simulink model "active_suspension"  (R2017a)
settings: Solver=VariableStepAuto  StartTime=0.0  StopTime=10.0  RelTol=1e-3
values from neighbouring files (symbols this model uses):
  A = z^2+den{1}(2)*z + den{1}(3)    [abs_spring18.m]    (also in active_suspension_ss.m = [0                 1                0                     0; active_suspension_ss_R.m = [0                 1                0                     0; active_suspension_ss_spring18.m = [0                 1                0                     0; double_integrator_deadbeat.m = [0 1; 0 0])
  B = num{1}(1)*z^2 + num{1}(2)*z + num{1}(3)    [abs_spring18.m]    (also in active_suspension_ss.m = [0                 0; active_suspension_ss_R.m = [0                 0; active_suspension_ss_spring18.m = [0                 0; double_integrator_deadbeat.m = [0;1])
  h = 0.05    [BLDC_partial2_fall18.m]    (also in abs_spring18.m = 0.2; active_suspension_ss.m = 0.00416985950901; active_suspension_ss_R.m = 0.00416985950901; active_suspension_ss_spring18.m = 0.004)
  L = acker(Phi, Gamma_u, p_d)    [active_suspension_ss_spring18.m]    (also in double_integrator_deadbeat.m = L'; final_dummy.m = Asf\bsf; hw_tank_simulink_pid_tuning.m = 2.84722131148; maglev_ss_partial2_spring18.m = place(A, B, pc))
undefined symbols (not defined in the file or in its folder): Lsh
settings Model: Creator=kjartan  LastModifiedBy=kjartan

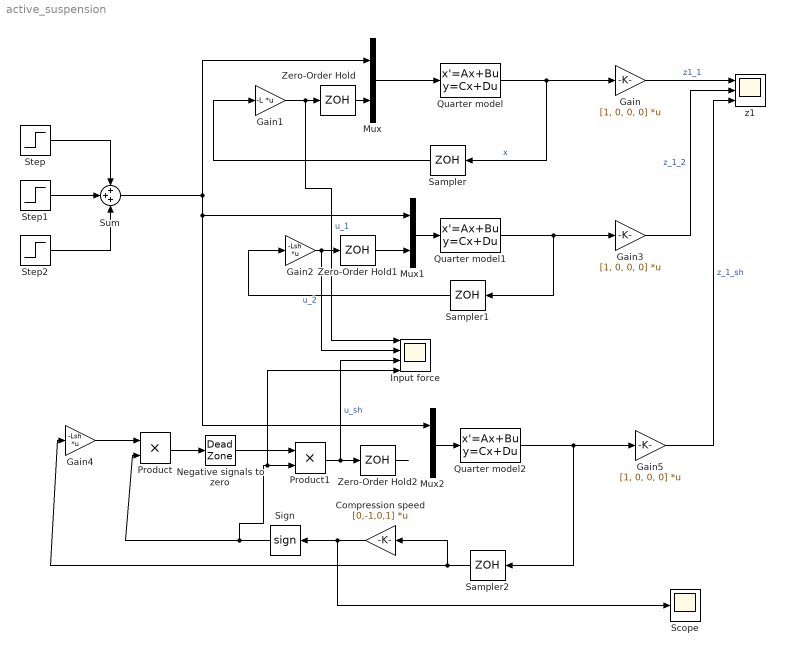
== system active_suspension ==
  Compression speed : Gain  Gain=[0,-1,0,1]  Multiplication=Matrix(K*u)
  Gain : Gain  Gain=[1, 0, 0, 0]  Multiplication=Matrix(K*u)
  Gain1 : Gain  Gain=-L  Multiplication=Matrix(K*u)
  Gain2 : Gain  Gain=-Lsh  Multiplication=Matrix(K*u)
  Gain3 : Gain  Gain=[1, 0, 0, 0]  Multiplication=Matrix(K*u)
  Gain4 : Gain  Gain=-Lsh  Multiplication=Matrix(K*u)
  Gain5 : Gain  Gain=[1, 0, 0, 0]  Multiplication=Matrix(K*u)
  Input force : Scope  NumInputPorts=4
  Mux : Mux  Inputs=2
  Mux1 : Mux  Inputs=2
  Mux2 : Mux  Inputs=2
  Negative signals to zero : DeadZone  LowerValue=-1e10  UpperValue=0  SaturateOnIntegerOverflow=on
  Product : Product
  Product1 : Product
  Quarter model : StateSpace  A=A  B=B  C=eye(4)  D=zeros(4,2)  X0=0
  Quarter model1 : StateSpace  A=A  B=B  C=eye(4)  D=zeros(4,2)  X0=0
  Quarter model2 : StateSpace  A=A  B=B  C=eye(4)  D=zeros(4,2)  X0=0
  Sampler : ZeroOrderHold  SampleTime=h
  Sampler1 : ZeroOrderHold  SampleTime=h
  Sampler2 : ZeroOrderHold  SampleTime=h
  Scope : Scope
  Sign : Signum
  Step : Step  After=0.1  SampleTime=0
  Step1 : Step  Time=2  After=-0.2  SampleTime=0
  Step2 : Step  Time=3  After=0.1  SampleTime=0
  Sum : Sum  Inputs=+++
  Zero-Order Hold : ZeroOrderHold  SampleTime=h
  Zero-Order Hold1 : ZeroOrderHold  SampleTime=h
  Zero-Order Hold2 : ZeroOrderHold  SampleTime=h
  z1 : Scope  NumInputPorts=3
  wires:
  Quarter model/1 -> Sampler/1, Gain/1  "x"
  Gain/1 -> z1/1  "z1_1"
  Mux/1 -> Quarter model/1
  Gain1/1 -> Input force/1, Zero-Order Hold/1  "u_1"
  Step/1 -> Sum/1
  Step1/1 -> Sum/2
  Step2/1 -> Sum/3
  Mux1/1 -> Quarter model1/1
  Gain2/1 -> Input force/2, Zero-Order Hold1/1  "u_2"
  Quarter model1/1 -> Sampler1/1, Gain3/1
  Gain3/1 -> z1/2  "z_1_2"
  Zero-Order Hold/1 -> Mux/2
  Sampler/1 -> Gain1/1
  Zero-Order Hold1/1 -> Mux1/2
  Sampler1/1 -> Gain2/1
  Sum/1 -> Mux/1, Mux2/1, Mux1/1
  Gain5/1 -> z1/3  "z_1_sh"
  Mux2/1 -> Quarter model2/1
  Sampler2/1 -> Compression speed/1, Gain4/1
  Quarter model2/1 -> Sampler2/1, Gain5/1
  Zero-Order Hold2/1 -> ?
  Gain4/1 -> Product/1
  Compression speed/1 -> Scope/1, Sign/1
  Sign/1 -> Input force/4, Product1/2, Product/2
  Product/1 -> Negative signals to zero/1
  Negative signals to zero/1 -> Product1/1
  Product1/1 -> Input force/3, Zero-Order Hold2/1  "u_sh"
